simulink model "Neurofeeedback_Fuzzy_without_fNIRS"  (R2022a)
settings: Solver=VariableStepAuto  StartTime=0.0  StopTime=50  RelTol=1e-3
libraries: fuzblock x1
settings Model: Creator=mariodelossantos  LastModifiedBy=mariodelossantos
settings DebuggingCC: UnconnectedInputMsg=warning  UnconnectedOutputMsg=warning  UnconnectedLineMsg=warning
settings RTWCC: DLArmComputeVersion=19.05

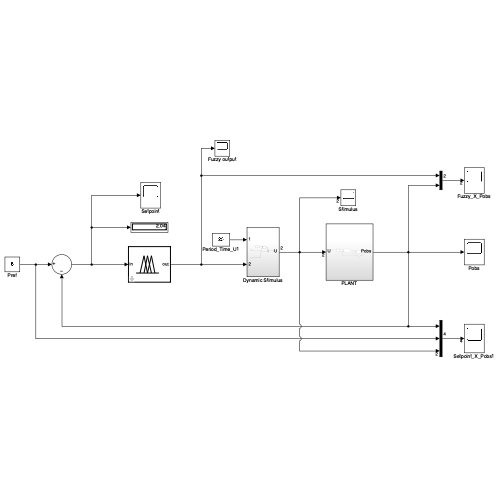
[thumbnail: Simulink's stored preview of the top-level diagram]
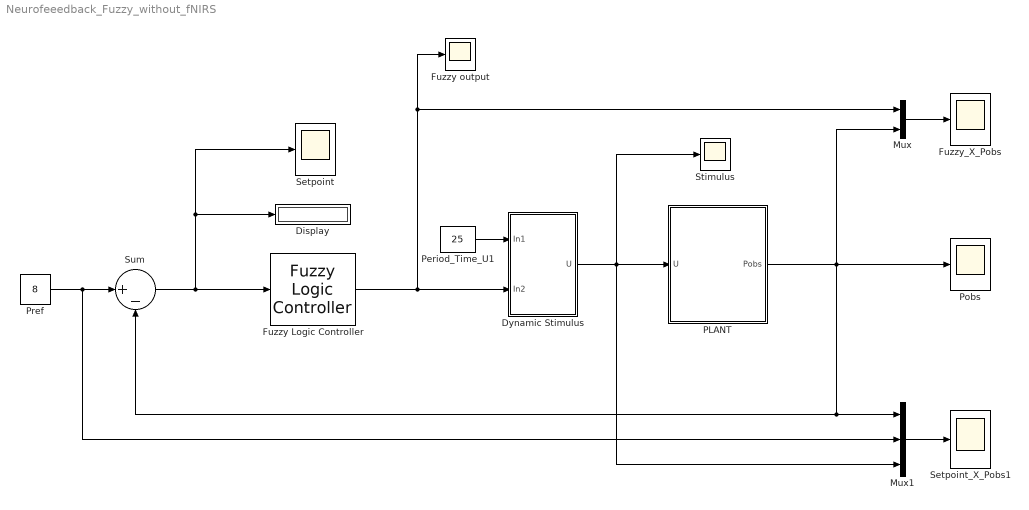
== system Neurofeeedback_Fuzzy_without_fNIRS ==
  Display : Display
  Dynamic Stimulus : Subsystem
  Fuzzy Logic Controller : fuzblock/Fuzzy Logic  Controller  FIS=cpWF  OutputSampleNumber=101  DataType=double  FuzzifiedInputs=off  RuleFiringStrengths=off  RuleOutputs=off  AggregatedOutputs=off  SimulateUsing=Interpreted execution  OutOfRangeInputValueMessage=warning  NoRuleFiredMessage=warning  EmptyOutputFuzzySetMessage=warning
  Fuzzy output : Scope
  Fuzzy_X_Pobs : Scope
  Mux : Mux  Inputs=2
  Mux1 : Mux  Inputs=3
  PLANT : Subsystem
  Period_Time_U1 : Constant  Value=25
  Pobs : Scope
  Pref : Constant  Value=8
  Setpoint : Scope
  Setpoint_X_Pobs1 : Scope
  Stimulus : Scope
  Sum : Sum  Inputs=|+-
  wires:
  PLANT/1(Pobs) -> Mux/2, Pobs/1, Mux1/1, Sum/2
  Fuzzy Logic Controller/1 -> Mux/1, Fuzzy output/1, Dynamic Stimulus/2(In2)
  Period_Time_U1/1 -> Dynamic Stimulus/1(In1)
  Dynamic Stimulus/1(U) -> Mux1/3, Stimulus/1, PLANT/1(U)
  Mux/1 -> Fuzzy_X_Pobs/1
  Mux1/1 -> Setpoint_X_Pobs1/1
  Pref/1 -> Mux1/2, Sum/1
  Sum/1 -> Fuzzy Logic Controller/1, Setpoint/1, Display/1

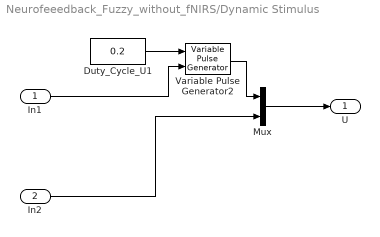
== system Neurofeeedback_Fuzzy_without_fNIRS/Dynamic Stimulus ==
  In1 : Inport
  In2 : Inport  Port=2
  Duty_Cycle_U1 : Constant  Value=0.2  OutMin=[0]  OutMax=[0.8]
  Mux : Mux  Inputs=2
  Variable Pulse Generator2 : VariablePulseGenerator  RunAtFixedTimeIntervals=on  SampleTime=1/10.4
  U : Outport
  wires:
  In1/1 -> Variable Pulse Generator2/2
  Mux/1 -> U/1
  Variable Pulse Generator2/1 -> Mux/1
  Duty_Cycle_U1/1 -> Variable Pulse Generator2/1
  In2/1 -> Mux/2

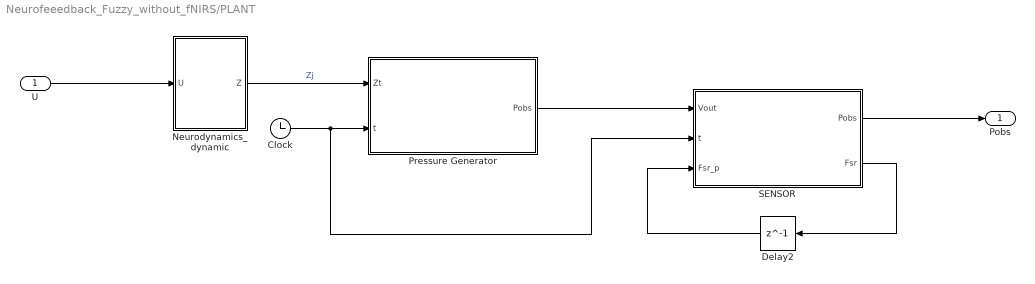
== system Neurofeeedback_Fuzzy_without_fNIRS/PLANT ==
  U : Inport
  Clock : Clock
  Delay2 : Delay  DelayLength=1  InitialCondition=0.0001
  Neurodynamics_dynamic : Subsystem
  Pressure Generator : MATLAB Function  TreatAsAtomicUnit=on
  SENSOR : MATLAB Function  TreatAsAtomicUnit=on
  Pobs : Outport
  wires:
  U/1 -> Neurodynamics_dynamic/1(U)
  Delay2/1 -> SENSOR/3(Fsr_p)
  SENSOR/2(Fsr) -> Delay2/1
  Clock/1 -> Pressure Generator/2(t), SENSOR/2(t)
  SENSOR/1(Pobs) -> Pobs/1
  Pressure Generator/1(Pobs) -> SENSOR/1(Vout)
  Neurodynamics_dynamic/1(Z) -> Pressure Generator/1(Zt)  "Zj"

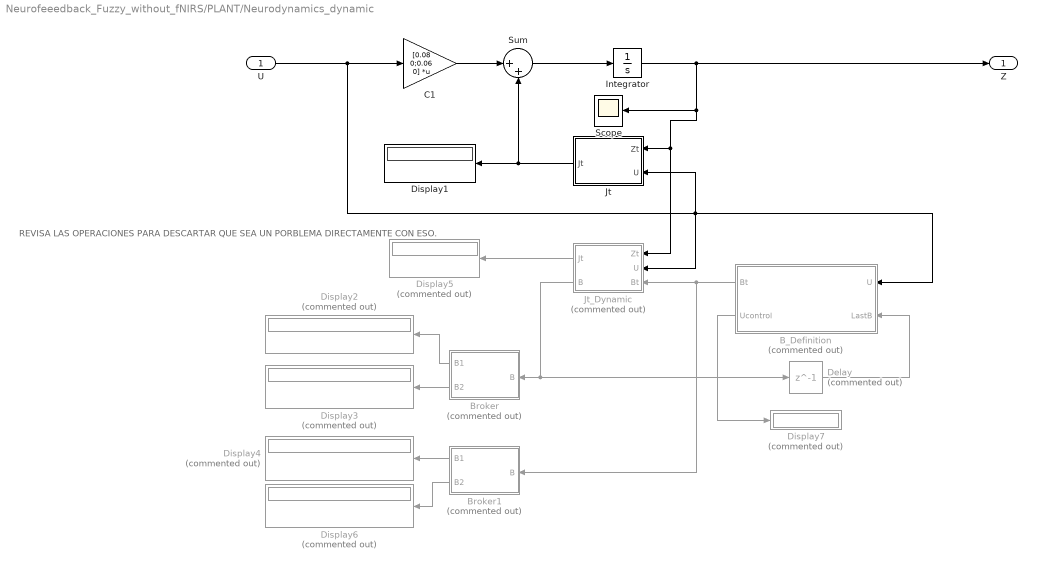
== system Neurofeeedback_Fuzzy_without_fNIRS/PLANT/Neurodynamics_dynamic ==
  note: REVISA LAS OPERACIONES PARA DESCARTAR QUE SEA UN PORBLEMA DIRECTAMENTE CON ESO.
  U : Inport
  B_Definition : MATLAB Function  Commented=on  TreatAsAtomicUnit=on
  Broker : MATLAB Function  Commented=on  TreatAsAtomicUnit=on
  Broker1 : MATLAB Function  Commented=on  TreatAsAtomicUnit=on
  C1 : Gain  Gain=[0.08 0;0.06 0]  Multiplication=Matrix(K*u)
  Delay : Delay  Commented=on  DelayLength=1  InitialCondition=0
  Display1 : Display
  Display{2..7} (6 alike) : Display  Commented=on
  Integrator : Integrator
  Jt : MATLAB Function  TreatAsAtomicUnit=on
  Jt_Dynamic : MATLAB Function  Commented=on  TreatAsAtomicUnit=on
  Scope : Scope
  Sum : Sum  Inputs=|++
  Z : Outport
  wires:
  Integrator/1 -> Z/1, Scope/1, Jt/1(Zt), Jt_Dynamic/1(Zt)
  C1/1 -> Sum/1
  U/1 -> C1/1, Jt/2(U), B_Definition/1(U), Jt_Dynamic/2(U)
  Jt_Dynamic/1(Jt) -> Display5/1
  Delay/1 -> B_Definition/2(LastB)
  Jt_Dynamic/2(B) -> Broker/1(B), Delay/1
  Broker/1(B1) -> Display2/1
  Broker/2(B2) -> Display3/1
  B_Definition/1(Bt) -> Broker1/1(B), Jt_Dynamic/3(Bt)
  Broker1/2(B2) -> Display6/1
  Broker1/1(B1) -> Display4/1
  B_Definition/2(Ucontrol) -> Display7/1
  Sum/1 -> Integrator/1
  Jt/1(Jt) -> Sum/2, Display1/1

== matlab function Neurofeeedback_Fuzzy_without_fNIRS/PLANT/SENSOR ==
  data: Vout input; Pobs output; t input; Fsr_p input; Fsr output
function [Pobs,Fsr] = PressureGenerator_sensor(Vout, t,Fsr_p)

    Vcc = 50; %Considering 5V as a real sensor, the value is on mV
    Rf = 100; %Fixed resistor 10k ohms
    kgf = 0.1019716213; % 1N = 0.1019716213 kgf
    Fsr = 0;
    Fsrforce = 0;
  
    Fsr = (Vcc - Vout * Rf) / Vout;
    FsConductance = 1000000; %Sensor conductance in uOhms
    FsConductance = FsConductance / Fsr;
    if FsConductance <= 1000
        Fsrforce = FsConductance / 80; %Force on Newtons
    else
        Fsrforce = FsConductance - 1000;
        Fsrforce = Fsrforce / 30;
    end
    
temp = Fsrforce * kgf;

Pobs = temp(1);

end

== matlab function Neurofeeedback_Fuzzy_without_fNIRS/PLANT/Pressure Generator ==
  data: Zt input; Pobs output; t input
function Pobs  = fcn(Zt, t)
    R=1000; %Resistor [Ohms];
    C= 2; %Capacitor [Faradays];
    V= Zt(1); %Voltage or system reference;
    Vc = V * (exp(-t/(R*C))); % Voltage at the capacitor  
    
Pobs = Vc;

== matlab function Neurofeeedback_Fuzzy_without_fNIRS/PLANT/Neurodynamics_dynamic/Broker ==
  data: B input; B1 output; B2 output
function [B1, B2] = fcn(B)
B1 = B(:,:,1);
B2 = B(:,:,2);

== matlab function Neurofeeedback_Fuzzy_without_fNIRS/PLANT/Neurodynamics_dynamic/Broker1 ==
  data: B input; B1 output; B2 output
function [B1, B2] = fcn(B)
B1 = B(:,:,1);
B2 = B(:,:,2);

== matlab function Neurofeeedback_Fuzzy_without_fNIRS/PLANT/Neurodynamics_dynamic/Jt_Dynamic ==
  data: Zt input; U input; Jt output; Bt input; B output
function [Jt, B] = fcn(Zt, U, Bt)

   A = [-0.16 -0.49;-0.02 -0.33];
   nRegions  = size(A,1);

   B = zeros(2,2,2);
   a = 0;
   B1 = [0 0; 0 0]; %There must be a B per stimulus
   B2 = [-0.02 -0.77; 0.33 -1.31];

   if Bt(:,:,2) ~= B(:,:,2)
       B(:,:,:) = Bt(:,:,:);
   else
          B(:,:,1) = B1;
          B(:,:,2) = B2;
   end
   M = size(U,1); %nStimuli
   assert(M == size(B,3),...
        'Unexpected number of induced connectivity parameters B.');

    simulationLength = size(U,2);
    for t = 1:simulationLength
       T = zeros(nRegions); %nRegions x nRegions
                   for uu = 1:M % Sum (Uj * Bj)
                       tmp = U(uu,t) * B(:,:,uu);
                       T = -0.5 * exp(T + tmp);  
                   end
            SI = diag(A);
    end
        A =  A - diag(exp(SI) + (SI));
Jt = (A*Zt) + (T*Zt);

== matlab function Neurofeeedback_Fuzzy_without_fNIRS/PLANT/Neurodynamics_dynamic/B_Definition ==
  settings: updateMethod=DISCRETE
  data: U input; Bt output; LastB input; Ucontrol output
function [Bt, Ucontrol] = B_Definition(U, LastB)
    Bt = zeros(2, 2, 2);
   %Control extraction and weight
   Ucontrol = U(2) * (0.1 + rand(1) * (1-0.1));
   Threshold = 0.1;
    if(Ucontrol < Threshold) %Random Ucontrol to test
        min = -1.5; 
        max =0.5;
        n = 2;
        r1 = min + rand(n)*(max-min);
        r2 = min + rand(n)*(max-min);
        %Bt(:,:,1) = r1(:,:);
        Bt(:,:,2) = r2(:,:);
    else
       Bt = LastB;
    end

== matlab function Neurofeeedback_Fuzzy_without_fNIRS/PLANT/Neurodynamics_dynamic/Jt ==
  data: Zt input; U input; Jt output
function Jt = fcn(Zt, U)
   A = [-0.16 -0.49;-0.02 -0.33];
   nRegions  = size(A,1);
   M = size(U,1); %nStimuli
   simulationLength = size(U,2);
   B = zeros(2,2,2);
   B1 = [0 0; 0 0]; %There must be a B per stimulus
   B2 = [-0.02 -0.77;
       0.33 -1.31];
   B(:,:,1) = B1;
   B(:,:,2) = B2;
      assert(M == size(B,3),...
       'Unexpected number of induced connectivity parameters B.');
   T = zeros(nRegions); %nRegions x nRegions
    for t = 1:simulationLength
           for uu = 1:M % Sum (Uj * Bj)
               tmp = U(uu,t)*B(:,:,uu);
               T = -0.5*exp(T + tmp);  
           end
    end
    SI = diag(A);
    A =  A - diag(exp(SI) + (SI));
Jt = (A*Zt) + (T*Zt);
